simulink model "model_integrator_proportional_regulator"  (R2019b)
settings: Solver=VariableStepAuto  StartTime=0.0  StopTime=1  RelTol=1e-3
settings Model: Creator=szymo  LastModifiedBy=szymo

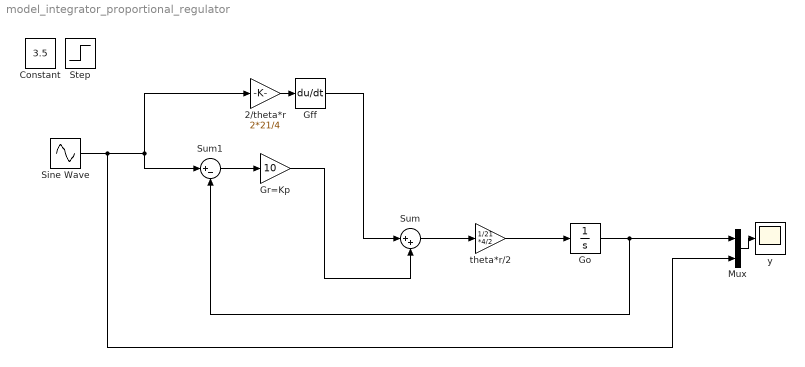
== system model_integrator_proportional_regulator ==
  2/theta*r : Gain  Gain=2*21/4
  Constant : Constant  Value=3.5
  Gff : Derivative
  Go : Integrator
  Gr=Kp : Gain  Gain=10
  Mux : Mux  Inputs=2
  Sine Wave : Sin  Amplitude=2  Frequency=50  SampleTime=0
  Step : Step  SampleTime=0
  Sum : Sum  Inputs=|++
  Sum1 : Sum  Inputs=|+-
  theta*r/2 : Gain  Gain=1/21 *4/2
  y : Scope
  wires:
  Go/1 -> Mux/1, Sum1/2
  theta*r/2/1 -> Go/1
  Sum/1 -> theta*r/2/1
  Gr=Kp/1 -> Sum/2
  Gff/1 -> Sum/1
  2/theta*r/1 -> Gff/1
  Sum1/1 -> Gr=Kp/1
  Sine Wave/1 -> Mux/2, Sum1/1, 2/theta*r/1
  Mux/1 -> y/1
